simulink model "Modulation"  (Simulink 7.8)
settings: Solver=ode4  StartTime=0.0  StopTime=80e-3  FixedStep=1e-6  RelTol=1e-3
libraries: simulink x1
settings Model: Creator=Daniel Montesinos  LastModifiedBy=Daniel Montesinos
settings OptimizationCC: InitFltsAndDblsToZero=on
settings DebuggingCC: SaveWithParameterizedLinksMsg=none  SignalResolutionControl=TryResolveAllWithWarning  MultiTaskDSMMsg=warning  MultiTaskCondExecSysMsg=none  FcnCallInpInsideContextMsg=Use local settings  StrictBusMsg=Warning
settings RTWCC: IncludeERTFirstTime=on
settings GRTTargetCC: TargetFcnLib=ansi_tfl_tmw.mat

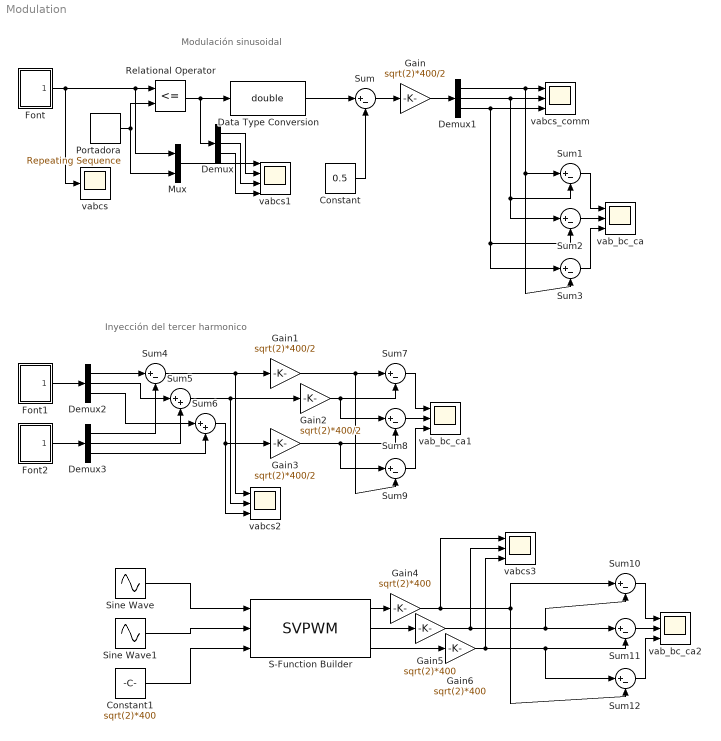
== system Modulation ==
  note: Modulación sinusoidal
  note: Inyección del tercer harmonico
  Constant : Constant  Value=0.5
  Constant1 : Constant  Value=sqrt(2)*400
  Data Type Conversion : DataTypeConversion  OutDataTypeStr=double
  Demux{,1..3} (4 alike) : Demux  Outputs=3
  Font : Subsystem
  Font1 : Subsystem
  Font2 : Subsystem
  Gain{,1..3} (4 alike) : Gain  Gain=sqrt(2)*400/2
  Gain4 : Gain  Gain=sqrt(2)*400
  Gain5 : Gain  Gain=sqrt(2)*400
  Gain6 : Gain  Gain=sqrt(2)*400
  Mux : Mux  Inputs=2
  Portadora : simulink/Sources/Repeating Sequence  rep_seq_t=[0 0.5e-3 1e-3]  rep_seq_y=[-1 1 -1]
  Relational Operator : RelationalOperator  Operator=<=  OutDataTypeStr=boolean
  S-Function Builder : S-Function  InitFcn=try, set_param(gcb,'FunctionName','SVPWM'), end  FunctionName=SVPWM  SFunctionModules=SVPWM_wrapper sign  WizardData=DataTag0  EnableBusSupport=off  mask(S-Function Builder){}
      mask init:
      | val = [[.9  0.75 0.75 1 1 .9 .9 1]',[1 1 0.75 0.75 .9 .9 1 .9]'];try , sys = get_param(gcb,'SfunBuilderFcnName');if isempty(sys), sys = get_param(gcb,'FunctionName'); end,catch, sys = get_param(gcb,'FunctionName'); end
      settings: CopyFcn=set_param(gcbh,'LinkStatus','none')  PreSaveFcn=try, set_param(gcb,'FunctionName','SVPWM'), end  OpenFcn=sfunctionwizard(gcbh)
      mask Display: plot(val(:,1),val(:,2)),disp(sys), port_label('input',1,'vsD'), port_label('input',2,'vsQ'), port_label('input',3,'VDC'), port_label('output',1,'duty_a'), port_label('output',2,'duty_b'), port_label('output',3,'duty_c')
  Sine Wave : Sin  Amplitude=sqrt(2)*230  Frequency=2*pi*50  Phase=pi/2  SampleTime=0
  Sine Wave1 : Sin  Amplitude=sqrt(2)*230  Frequency=2*pi*50  SampleTime=0
  Sum{,1..4,7..12} (11 alike) : Sum  Inputs=|+-
  Sum5 : Sum  Inputs=|++
  Sum6 : Sum  Inputs=|++
  vab_bc_ca : Scope  NumInputPorts=3
      settings: YMin=-300~-300~-300  YMax=300~300~300  SaveName=ScopeData2
  vab_bc_ca1 : Scope  NumInputPorts=3
      settings: YMin=-750~-750~-750  YMax=750~750~750  SaveName=ScopeData4
  vab_bc_ca2 : Scope  NumInputPorts=3
      settings: YMin=-750~-750~-750  YMax=750~750~750  SaveName=ScopeData6
  vabcs : Scope
  vabcs1 : Scope  NumInputPorts=4
      settings: YMin=-5~-5~-5~-5  YMax=5~5~5~5  SaveName=PWM
  vabcs2 : Scope  NumInputPorts=3
      settings: YMin=-1.5~-1.25~-1.25  YMax=1.5~1.25~1.25  SaveName=ScopeData3
  vabcs3 : Scope  NumInputPorts=3
      settings: YMin=-300~-300~-300  YMax=300~300~300  SaveName=ScopeData5
  vabcs_comm : Scope  NumInputPorts=3
      settings: YMin=-5~-5~-5  YMax=5~5~5
  wires:
  Font/1(vabcs) -> vabcs/1, Relational Operator/1, Mux/1
  Portadora/1 -> Relational Operator/2, Mux/2
  Relational Operator/1 -> Demux/1, Data Type Conversion/1
  Mux/1 -> vabcs1/1
  Data Type Conversion/1 -> Sum/1
  Constant/1 -> Sum/2
  Sum/1 -> Gain/1
  Gain/1 -> Demux1/1
  Demux1/1 -> vabcs_comm/1, Sum1/1, Sum3/2
  Demux1/2 -> vabcs_comm/2, Sum1/2, Sum2/1
  Demux1/3 -> vabcs_comm/3, Sum2/2, Sum3/1
  Sum1/1 -> vab_bc_ca/1
  Sum2/1 -> vab_bc_ca/2
  Sum3/1 -> vab_bc_ca/3
  Demux/1 -> vabcs1/2
  Demux/2 -> vabcs1/3
  Demux/3 -> vabcs1/4
  Font1/1(vabcs) -> Demux2/1
  Font2/1(vabcs) -> Demux3/1
  Demux2/1 -> Sum4/1
  Demux3/1 -> Sum4/2
  Demux2/2 -> Sum5/1
  Demux2/3 -> Sum6/1
  Demux3/2 -> Sum5/2
  Demux3/3 -> Sum6/2
  Sum4/1 -> vabcs2/1, Gain1/1
  Sum5/1 -> vabcs2/2, Gain2/1
  Sum6/1 -> vabcs2/3, Gain3/1
  Sum7/1 -> vab_bc_ca1/1
  Sum8/1 -> vab_bc_ca1/2
  Sum9/1 -> vab_bc_ca1/3
  Gain1/1 -> Sum7/1, Sum9/2
  Gain2/1 -> Sum7/2, Sum8/1
  Gain3/1 -> Sum8/2, Sum9/1
  Sine Wave/1 -> S-Function Builder/1
  Sine Wave1/1 -> S-Function Builder/2
  Constant1/1 -> S-Function Builder/3
  S-Function Builder/1 -> Gain4/1
  S-Function Builder/2 -> Gain5/1
  S-Function Builder/3 -> Gain6/1
  Sum10/1 -> vab_bc_ca2/1
  Sum11/1 -> vab_bc_ca2/2
  Sum12/1 -> vab_bc_ca2/3
  Gain4/1 -> Sum10/1, Sum12/2, vabcs3/1
  Gain5/1 -> Sum10/2, Sum11/1, vabcs3/2
  Gain6/1 -> Sum11/2, Sum12/1, vabcs3/3

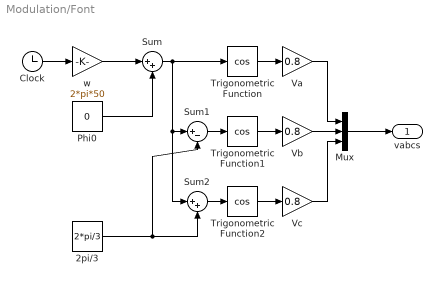
== system Modulation/Font ==
  2pi/3 : Constant  Value=2*pi/3
  Clock : Clock
  Mux : Mux  Inputs=3
  Phi0 : Constant  Value=0
  Sum : Sum  Inputs=|++
  Sum1 : Sum  Inputs=|+-
  Sum2 : Sum  Inputs=|++
  Trigonometric Function : Trigonometry  Operator=cos
  Trigonometric Function1 : Trigonometry  Operator=cos
  Trigonometric Function2 : Trigonometry  Operator=cos
  Va : Gain  Gain=0.8
  Vb : Gain  Gain=0.8
  Vc : Gain  Gain=0.8
  w : Gain  Gain=2*pi*50
  vabcs : Outport
  wires:
  Clock/1 -> w/1
  w/1 -> Sum/1
  Phi0/1 -> Sum/2
  Sum/1 -> Trigonometric Function/1, Sum1/1, Sum2/1
  2pi/3/1 -> Sum2/2, Sum1/2
  Sum1/1 -> Trigonometric Function1/1
  Sum2/1 -> Trigonometric Function2/1
  Trigonometric Function/1 -> Va/1
  Trigonometric Function1/1 -> Vb/1
  Trigonometric Function2/1 -> Vc/1
  Mux/1 -> vabcs/1
  Va/1 -> Mux/1
  Vb/1 -> Mux/2
  Vc/1 -> Mux/3

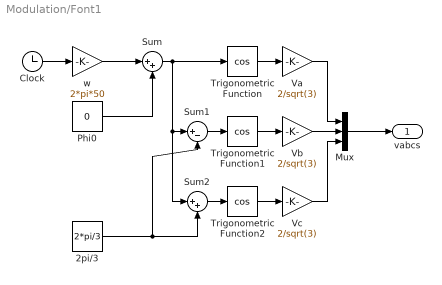
== system Modulation/Font1 ==
  2pi/3 : Constant  Value=2*pi/3
  Clock : Clock
  Mux : Mux  Inputs=3
  Phi0 : Constant  Value=0
  Sum : Sum  Inputs=|++
  Sum1 : Sum  Inputs=|+-
  Sum2 : Sum  Inputs=|++
  Trigonometric Function : Trigonometry  Operator=cos
  Trigonometric Function1 : Trigonometry  Operator=cos
  Trigonometric Function2 : Trigonometry  Operator=cos
  Va : Gain  Gain=2/sqrt(3)
  Vb : Gain  Gain=2/sqrt(3)
  Vc : Gain  Gain=2/sqrt(3)
  w : Gain  Gain=2*pi*50
  vabcs : Outport
  wires:
  Clock/1 -> w/1
  w/1 -> Sum/1
  Phi0/1 -> Sum/2
  Sum/1 -> Trigonometric Function/1, Sum1/1, Sum2/1
  2pi/3/1 -> Sum2/2, Sum1/2
  Sum1/1 -> Trigonometric Function1/1
  Sum2/1 -> Trigonometric Function2/1
  Trigonometric Function/1 -> Va/1
  Trigonometric Function1/1 -> Vb/1
  Trigonometric Function2/1 -> Vc/1
  Mux/1 -> vabcs/1
  Va/1 -> Mux/1
  Vb/1 -> Mux/2
  Vc/1 -> Mux/3

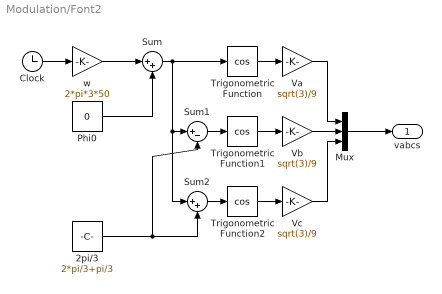
== system Modulation/Font2 ==
  2pi/3 : Constant  Value=2*pi/3+pi/3
  Clock : Clock
  Mux : Mux  Inputs=3
  Phi0 : Constant  Value=0
  Sum : Sum  Inputs=|++
  Sum1 : Sum  Inputs=|+-
  Sum2 : Sum  Inputs=|++
  Trigonometric Function : Trigonometry  Operator=cos
  Trigonometric Function1 : Trigonometry  Operator=cos
  Trigonometric Function2 : Trigonometry  Operator=cos
  Va : Gain  Gain=sqrt(3)/9
  Vb : Gain  Gain=sqrt(3)/9
  Vc : Gain  Gain=sqrt(3)/9
  w : Gain  Gain=2*pi*3*50
  vabcs : Outport
  wires:
  Clock/1 -> w/1
  w/1 -> Sum/1
  Phi0/1 -> Sum/2
  Sum/1 -> Trigonometric Function/1, Sum1/1, Sum2/1
  2pi/3/1 -> Sum2/2, Sum1/2
  Sum1/1 -> Trigonometric Function1/1
  Sum2/1 -> Trigonometric Function2/1
  Trigonometric Function/1 -> Va/1
  Trigonometric Function1/1 -> Vb/1
  Trigonometric Function2/1 -> Vc/1
  Mux/1 -> vabcs/1
  Va/1 -> Mux/1
  Vb/1 -> Mux/2
  Vc/1 -> Mux/3
